simulink library "Air_Resistance"  (R2018b)
settings: Solver=VariableStepAuto  StartTime=0.0  StopTime=10.0  RelTol=1e-3
settings Model: Creator=Alexander Koch  LastModifiedBy=ga69qig
settings SFSimCC: SimUseLocalCustomCode=off
settings RTWCC: RTWUseLocalCustomCode=off
settings CodeAppCC: StateflowObjectComments=on

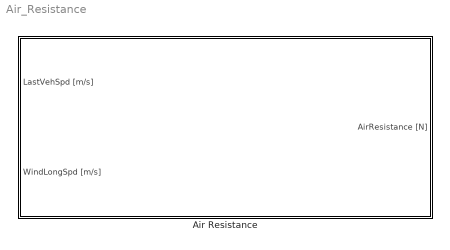
== system Air_Resistance ==
  Air Resistance : Subsystem  mask(SB){A_st=2, Roh_Air=1.19, c_w=0.3, LocalSampleTime=-1}
      mask prompts: A_st "Front Surface [m^2]"; Roh_Air "Density Air [kg/m^3]"; c_w "c_w-Factor [-]"; LocalSampleTime "Local System Sample-Time [s]"
      mask help:
      | <Author> Alexander Koch, Benedikt Danquah based on Stefan Müller [1], Stephan Rohr [2]  </Author>
      | <Date> 21/03/2017 </Date>
      | <Sources>
      | [1] S. Mueller, S. Rohr, und et al, Hrsg, Analysing the Influence of Driver Behaviour and Tuning Measures on Battery Aging and Residual Value of Electric Vehicles, 2017
      | </Sources>
      |
      | <Description>
      | Requires the last vehicle speed available, the longitudinal wind speed of the environment and the vehicle parameters front surface, air density and the c_w factor. Calculates the air drag in Newton.
      | </Description>
      mask init:
      | GlobalSampleTime = CalcGlobalSampleTime(LocalSampleTime);
      mask Help:
      | <Parameters>
      | Front Surface [m^2]
      | 	<Min> >0 </Min>
      | Density Air [kg/m^3]
      | 	<Min> 0 </Min>
      | c_w-Factor [-]
      | 	<Min> >0 </Min>
      | Local System Sample-Time [s]
      | 	<Min> GlobalSampleTime </Min>
      | Global Sample-Time [s]
      | </Parameters>
      | 
      | <Inputs>
      | LastVehSpd [m/s]
      | WindLongSpd [m/s]
      | 	<sign orientation> [+] tail wind </sign orientation>
      | </Inputs>
      | 
      | <Outputs>
      | AirResistance [N]
      | 	<sign orientation> [+] drag </sign orientation>
      | </Outputs>
      | <Sources>
      | [1] S. Mueller, S. Rohr, W. Schmid, and M. Lienkamp, “Analysing the Influence of Driver Behaviour and Tuning Measures on Battery Aging and Residual Value of Electric Vehicles,” in Proc. EVS30 Symposium, Stuttgart, 2017, pp. 1–12.
      | [2] S. Rohr, “Technisch-wirtschaftliche Analyse des Zweitnutzungs- potentials von Lithium-Ionen-Traktionsbatterien,” Dissertation, Institute of Automotive Technology, Technical University Munich, Munich, 2018.
      | </Sources>
      mask TypeOptions A_st: A_St [m]/Value
      mask TypeOptions Roh_Air: Roh_Air [kg//m3]/Value
      mask TypeOptions c_w: c_w/Value
      mask TypeOptions LocalSampleTime: LastVehSpd [m//s]/SampleTime | WindLongSpd [m//s]/SampleTime
      mask DialogControl Container3 Prompt: Documentation:
      mask DialogControl Control2 Prompt: %<MaskHelp>
      mask DialogControl Container5 Prompt: Sample Time
      mask Display:
      | [picturexpos,pictureypos,picturewidth,pictureheight] = ...
      |     CalcBlockPicturePosition(gcb,8.5/6.5,0.01,0.1,100,100); % calculating picture position depending on Block size and minimum margin size
      | image('Air_Resistance.svg',[picturexpos pictureypos picturewidth pictureheight]); % plot picture to block

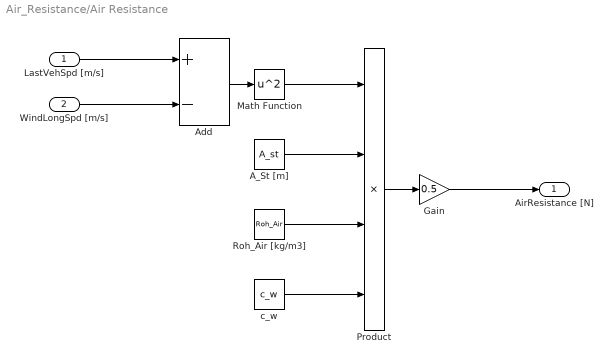
== system Air_Resistance/Air Resistance ==
  LastVehSpd [m/s] : Inport  SampleTime=LocalSampleTime
  WindLongSpd [m/s] : Inport  Port=2  SampleTime=LocalSampleTime
  A_St [m] : Constant  Value=A_st
  Add : Sum  Inputs=+-
  Gain : Gain  Gain=0.5
  Math Function : Math  Operator=square  SaturateOnIntegerOverflow=on
  Product : Product  Inputs=4
  Roh_Air [kg/m3] : Constant  Value=Roh_Air
  c_w : Constant  Value=c_w
  AirResistance [N] : Outport  SampleTime=GlobalSampleTime
  wires:
  Gain/1 -> AirResistance [N]/1
  Roh_Air [kg/m3]/1 -> Product/3
  A_St [m]/1 -> Product/2
  Math Function/1 -> Product/1
  Product/1 -> Gain/1
  WindLongSpd [m/s]/1 -> Add/2
  LastVehSpd [m/s]/1 -> Add/1
  c_w/1 -> Product/4
  Add/1 -> Math Function/1
